simulink library "fuselagePool_cl"  (R2020a)
settings: Solver=VariableStepAuto  StartTime=0.0  StopTime=10.0  RelTol=1e-3
undefined symbols (not defined in the file): fuse, rho, vcl, vhcl
libraries: vrlib x2, dynamicPressure_ul x1, localApparentWind_ul x1
settings Model: Creator=mcobb  LastModifiedBy=adabney
settings DataIOCC: ReturnWorkspaceOutputs=off
settings DebuggingCC: ArithmeticOperatorsInVariantConditions=warning
settings SFSimCC: CustomCodeUndefinedFunction=UseInterfaceOnly

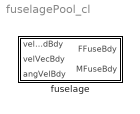
== system fuselagePool_cl ==
  fuselage : Subsystem  mask{momArm=vcl.fuseMomentArm.Value, fus=vcl.fuse, fusRhoDa=rho}
      mask prompts: momArm "Fuselage Moment Arm"; fus "Fuselage"; fusRhoDa "Density"
      mask DialogControl Container4 Prompt: General
      mask DialogControl Container9 Prompt: Fuselage object (OCT.fuselage)
      mask DialogControl Container8 Prompt: Environment Object (OCT.env)

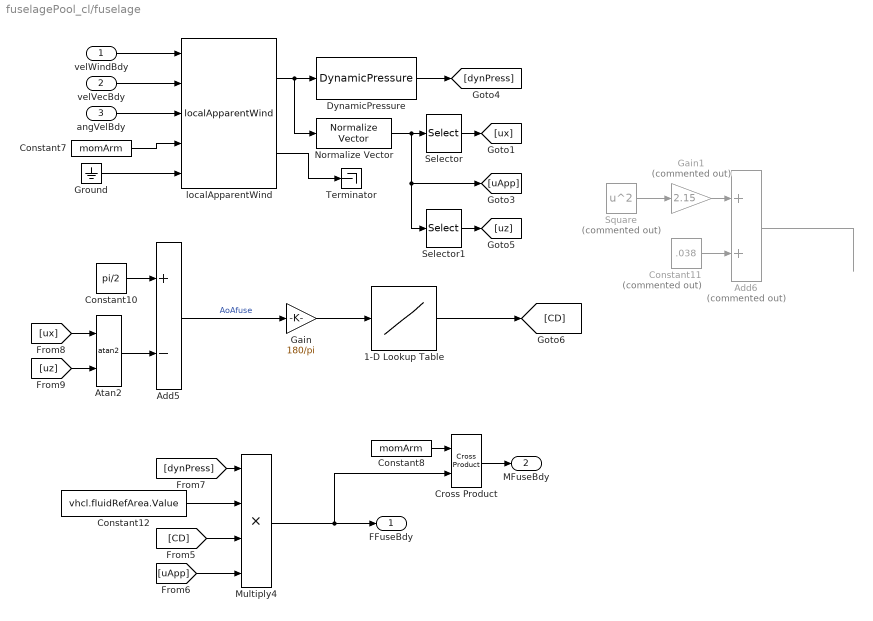
== system fuselagePool_cl/fuselage ==
  velWindBdy : Inport
  velVecBdy : Inport  Port=2
  angVelBdy : Inport  Port=3
  1-D Lookup Table : Lookup_n-D  NumberOfTableDimensions=1  BreakpointsForDimension1=fus.alpha.Value  Table=fuse.CD.Value  InternalRulePriority=Speed  RndMeth=Simplest  InputSameDT=on
  Add5 : Sum  Inputs=+-
  Add6 : Sum  Commented=on
  Atan2 : Trigonometry  Operator=atan2
  Constant10 : Constant  Value=pi/2
  Constant11 : Constant  Commented=on  Value=.038
  Constant12 : Constant  Value=vhcl.fluidRefArea.Value
  Constant7 : Constant  Value=momArm
  Constant8 : Constant  Value=momArm
  Cross Product : vrlib/Utilities/Cross Product
  DynamicPressure : dynamicPressure_ul/DynamicPressure  rho=fusRhoDa
  Gain : Gain  Gain=180/pi
  Gain1 : Gain  Commented=on  Gain=2.15
  Ground : Ground
  Multiply4 : Product  Inputs=4
  Normalize Vector : vrlib/Utilities/Normalize Vector  maxzero=0
  Selector : Selector  InputPortWidth=3  IndexOptions=Index vector (dialog)  Indices=1  OutputSizes=1
  Selector1 : Selector  InputPortWidth=3  IndexOptions=Index vector (dialog)  Indices=3  OutputSizes=1
  Square : Math  Commented=on  Operator=square  SaturateOnIntegerOverflow=on
  Terminator : Terminator
  localApparentWind : localApparentWind_ul/localApparentWind  SystemSampleTime=-1  Latency=0  AutoFrameSizeCalculation=off
  FFuseBdy : Outport  VectorParamsAs1DForOutWhenUnconnected=off
  MFuseBdy : Outport  Port=2  VectorParamsAs1DForOutWhenUnconnected=off
  wires:
  Cross Product/1 -> MFuseBdy/1
  Constant8/1 -> Cross Product/1
  DynamicPressure/1 -> [dynPress]
  velWindBdy/1 -> localApparentWind/1
  Constant7/1 -> localApparentWind/4
  velVecBdy/1 -> localApparentWind/2
  localApparentWind/1 -> Normalize Vector/1, DynamicPressure/1
  angVelBdy/1 -> localApparentWind/3
  [uApp] -> Multiply4/4
  [CD] -> Multiply4/3
  Constant12/1 -> Multiply4/2
  [dynPress] -> Multiply4/1
  Multiply4/1 -> FFuseBdy/1, Cross Product/2
  Selector/1 -> [ux]
  Normalize Vector/1 -> Selector/1, Selector1/1, [uApp]
  Ground/1 -> localApparentWind/5
  localApparentWind/2 -> Terminator/1
  Selector1/1 -> [uz]
  [ux] -> Atan2/1
  [uz] -> Atan2/2
  Constant10/1 -> Add5/1
  Atan2/1 -> Add5/2
  Add5/1 -> Gain/1  "AoAfuse"
  Square/1 -> Gain1/1
  Constant11/1 -> Add6/2
  Gain1/1 -> Add6/1
  Add6/1 -> ?
  Gain/1 -> 1-D Lookup Table/1
  1-D Lookup Table/1 -> [CD]
